simulink model "motor_stepper"  (R2018b)
settings: Solver=VariableStepAuto  StartTime=0.0  StopTime=2  FixedStep=0.001  MaxStep=0.001  RelTol=1e-3  EnableMultiTasking=on
libraries: fl_lib x27, nesl_utility x6, elec_lib x2, simulink x1
CloseFcn:
  | try,close(h1_elec_motor_stepper),end
  | clear h1_elec_motor_stepper
  | try,close(h2_elec_motor_stepper),end
  | clear h2_elec_motor_stepper
  | 
  | clear simlog_elec_motor_stepper
  | clear logsout_elec_motor_stepper
  | clear RPM2 tout
Description:
  | Stepper Motor with Control
  | 
  | Copyright 2008-2018 The MathWorks, Inc.
settings Model: Creator=MathWorks  LastModifiedBy=Administrator
settings DataIOCC: MaxDataPoints=10000  SaveFormat=Array  SignalLoggingName=logsout_elec_motor_stepper
settings OptimizationCC: ExpressionDepthLimit=2147483647  InitFltsAndDblsToZero=on  LifeSpan=inf
settings DebuggingCC: UnderspecifiedInitializationDetection=Classic  MergeDetectMultiDrivingBlocksExec=none  FcnCallInpInsideContextMsg=warning  StateNameClashWarn=warning  LibraryContextMissingDiagnostic=none  SFUnexpectedBacktrackingDiag=warning  SFNoUnconditionalDefaultTransitionDiag=warning  SFExecutionAtInitializationDiag=none
settings HardwareCC: ProdBitPerPointer=32  ProdBitPerSizeT=32  ProdBitPerPtrDiffT=32  ProdLargestAtomicFloat=None  ProdIntDivRoundTo=Undefined  ProdEndianess=Unspecified  ProdWordSize=32  ProdHWDeviceType=32-bit Generic
settings ModelReferenceCC: PropagateSignalLabelsOutOfModel=off
settings SFSimCC: SimUseLocalCustomCode=off
settings RTWCC: RTWUseLocalCustomCode=off
settings CodeAppCC: StateflowObjectComments=on
settings GRTTargetCC: TargetLangStandard=C89/C90 (ANSI)  GeneratePreprocessorConditionals=Disable all  CombineOutputUpdateFcns=off  GRTInterface=on
settings ConfigComp: CovScope=ReferencedModels  CovMetricSettings=dw  CovHtmlReporting=on  CovSaveCumulativeToWorkspaceVar=on  CovSaveSingleToWorkspaceVar=on  CovExternalEMLEnable=off  CovSFcnEnable=off
settings SimscapeCC: SimscapeLogType=all  SimscapeLogSimulationStatistics=on  SimscapeLogName=simlog_elec_motor_stepper  SimscapeLogDataHistory=10000

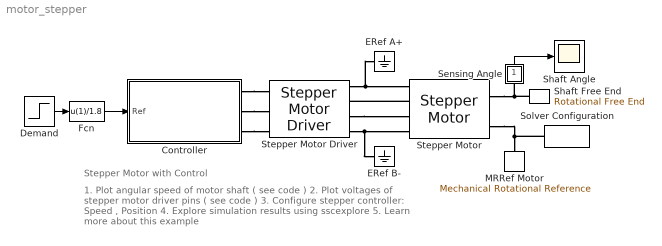
== system motor_stepper ==
  note: Stepper Motor with Control
  note: 1. Plot angular speed of motor shaft ( see code )
      | 2. Plot voltages of stepper motor driver pins ( see code )
      | 3. Configure stepper controller: Speed , Position
      | 4. Explore simulation results using sscexplore
      | 5. Learn more about this example
  Controller : Subsystem  VariantControlMode=Label  Variant=on  LabelModeActiveChoice=Position
      settings: AttributesFormatString=%<BlockChoice>
  Demand : Step  Before=10  After=0  SampleTime=0
  ERef A+ : fl_lib/Electrical/Electrical Elements/Electrical Reference
      settings: SourceProductName=Foundation Library
  ERef B- : fl_lib/Electrical/Electrical Elements/Electrical Reference
      settings: SourceProductName=Foundation Library
  Fcn : Fcn  Expr=u(1)/1.8
  MRRef Motor : fl_lib/Mechanical/Rotational Elements/Mechanical Rotational Reference
      settings: SourceProductName=Foundation Library
  Sensing Angle : Subsystem
      mask Display: disp('a')
  Shaft Angle : Scope
  Shaft Free End : fl_lib/Mechanical/Rotational Elements/Rotational Free End  w_specify=off  w_priority=None  w=0 rad/s  w_nominal_specify=off  w_nominal_unit=rad/s  w_nominal_value=1
      settings: SourceProductName=Foundation Library
  Solver Configuration : nesl_utility/Solver Configuration  PhysicalDomain=network_engine_domain  SubClassName=solver  LeftPortType=input  RightPortType=generic  Tones=[]  Harmonics=[]  SimulateNoise=off  Profile=off  UseLocalSampling=off  EnableSwitchedLinearOptims=on  FrequencyDomain=off  UseCCode=off  RelTol=0.001  AbsTol=1e-06  MinStep=1e-09  ToWorkspace=off  RevertToSquareIcSolve=off  NumHomotopyIterations=100  PhasorMode=off  PhasorModeNumHarmonics=1  DoDC=off  ResidualTolerance=1e-9  UseLocalSolver=off  LocalSolverChoice=NE_BACKWARD_EULER_ADVANCER  LocalSolverSampleTime=.001  DoFixedCost=off  MaxNonlinIter=3  MaxModeIter=2  LinearAlgebra=auto  EquationFormulation=NE_TIME_EF  DelaysMemoryBudget=1024  AutomaticFiltering=on  FilteringTimeConstant=0.001  PartitionStorageMethod=AS_NEEDED  PartitionMemoryBudget=1024
  Stepper Motor : elec_lib/Actuators & Drivers/Rotational Actuators/Stepper Motor  step_or_av=1  w_vec=[ 0 1000 3e+3 ] rpm  T_vec=[ 2 2 1 ] N*m  assert_if_slipping=0  J_total=1e-4 kg*m^2  max_step_rate=10 Hz  Ra=0.55 Ohm  La=0.0015 H  Km=0.19 N*m/A  Td=0 N*m  Rm=Inf Ohm  Step=1.8 deg  J=4.5e-05 kg*m^2  B=1e-02 N*m/(rad/s)  speed0=0 rpm  theta0=0 deg  alpha=[ 0.00393 0.00393 ] 1/K  Tmeas=25 degC  T_vec2=[ 1.7 1.7 0.85 ] N*m  Tmeas2=125 degC  half_stepping=0  thermal_masses=[ 100 100 ] J/K  initial_temperatures=[ 25 25 ] degC  rotor_thermal_mass=50 J/K  rotor_initial_temperature=25 degC  Rm_percent_rotor=90
      settings: SourceProductName=Simscape Electronics  SourceProductBaseCode=SN
  Stepper Motor Driver : elec_lib/Actuators & Drivers/Drivers/Stepper Motor Driver  step_or_av=1  step_rate_per_volt=10 Hz/V  Venable=2.5 V  Vreverse=2.5 V  Vm=5 V  half_stepping=0
      settings: SourceProductName=Simscape Electronics  SourceProductBaseCode=SN
  wires:
  Demand/1 -> Fcn/1
  Sensing Angle/1(theta) -> Shaft Angle/1
  Fcn/1 -> Controller/1(Ref)
  connections:
  Stepper Motor Driver/RConn1 -- Stepper Motor/LConn1 -- ERef A+/LConn1
  Stepper Motor/LConn2 -- Stepper Motor Driver/RConn2
  Stepper Motor Driver/RConn3 -- Stepper Motor/LConn3
  Stepper Motor Driver/RConn4 -- Stepper Motor/LConn4 -- ERef B-/LConn1
  Stepper Motor/RConn1 -- Shaft Free End/LConn1 -- Sensing Angle/LConn1
  Stepper Motor/RConn2 -- Solver Configuration/RConn1 -- MRRef Motor/LConn1
  Controller/RConn1 -- Stepper Motor Driver/LConn1
  Controller/RConn2 -- Stepper Motor Driver/LConn2
  Controller/RConn3 -- Stepper Motor Driver/LConn3

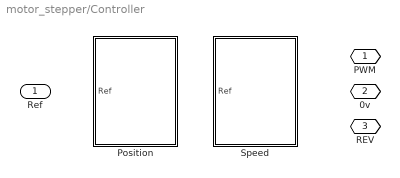
== system motor_stepper/Controller ==
  Ref : Inport
  Position : Subsystem  VariantControl=Position
  Speed : Subsystem  VariantControl=Speed
  PWM : PMIOPort  Side=Right
  0v : PMIOPort  Port=2  Side=Right
  REV : PMIOPort  Port=3  Side=Right

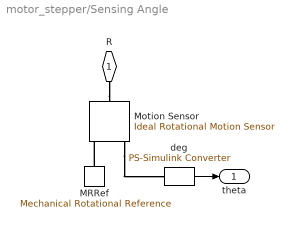
== system motor_stepper/Sensing Angle ==
  MRRef : fl_lib/Mechanical/Rotational Elements/Mechanical Rotational Reference
      settings: SourceProductName=Foundation Library
  Motion Sensor : fl_lib/Mechanical/Mechanical Sensors/Ideal Rotational Motion Sensor  offset=0 rad
      settings: SourceProductName=Foundation Library
  deg : nesl_utility/PS-Simulink Converter  PhysicalDomain=network_engine_domain  SubClassName=ps_output  LeftPortType=input  RightPortType=output  PseudoPeriodic=off  Frequencies=[]  Unit=deg  AffineConversion=off
  R : PMIOPort  Side=Left
  theta : Outport
  wires:
  deg/1 -> theta/1
  connections:
  R/RConn1 -- Motion Sensor/LConn1
  Motion Sensor/RConn3 -- deg/LConn1
  MRRef/LConn1 -- Motion Sensor/RConn1

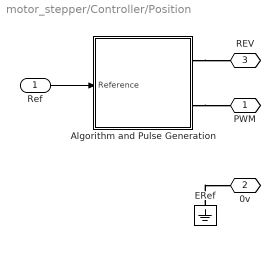
== system motor_stepper/Controller/Position ==
  Ref : Inport
  Algorithm and Pulse Generation : Subsystem
  ERef : fl_lib/Electrical/Electrical Elements/Electrical Reference
      settings: SourceProductName=Foundation Library
  PWM : PMIOPort  Side=Right
  0v : PMIOPort  Port=2  Side=Right
  REV : PMIOPort  Port=3  Side=Right
  wires:
  Ref/1 -> Algorithm and Pulse Generation/1(Reference)
  connections:
  Algorithm and Pulse Generation/RConn2 -- PWM/RConn1
  Algorithm and Pulse Generation/RConn1 -- REV/RConn1
  ERef/LConn1 -- 0v/RConn1

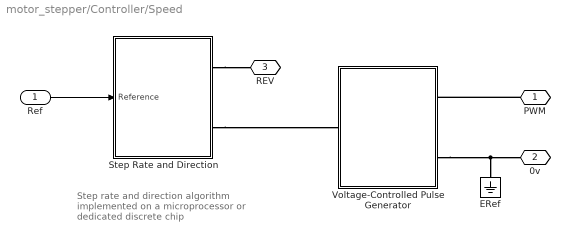
== system motor_stepper/Controller/Speed ==
  note: Step rate and direction algorithm implemented on a microprocessor or dedicated discrete chip
  Ref : Inport
  ERef : fl_lib/Electrical/Electrical Elements/Electrical Reference
      settings: SourceProductName=Foundation Library
  Step Rate and Direction : Subsystem
  Voltage-Controlled Pulse Generator : Subsystem
  PWM : PMIOPort  Side=Right
  0v : PMIOPort  Port=2  Side=Right
  REV : PMIOPort  Port=3  Side=Right
  wires:
  Ref/1 -> Step Rate and Direction/1(Reference)
  connections:
  PWM/RConn1 -- Voltage-Controlled Pulse Generator/RConn1
  Voltage-Controlled Pulse Generator/RConn2 -- 0v/RConn1 -- ERef/LConn1
  Step Rate and Direction/RConn1 -- REV/RConn1
  Step Rate and Direction/RConn2 -- Voltage-Controlled Pulse Generator/LConn1

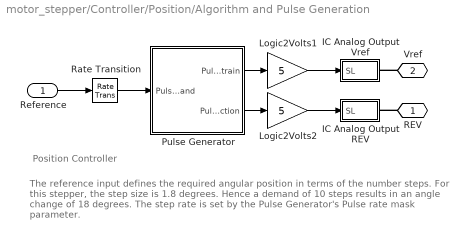
== system motor_stepper/Controller/Position/Algorithm and Pulse Generation ==
  note: The reference input defines the required angular position in terms of
      | the number steps. For this stepper, the step size is 1.8 degrees. Hence
      | a demand of 10 steps results in an angle change of 18 degrees.
      | The step rate is set by the Pulse Generator's Pulse rate mask parameter.
  note: Position Controller
  Reference : Inport
  IC Analog Output REV : Subsystem
  IC Analog Output Vref : Subsystem
  Logic2Volts1 : Gain  Gain=5
  Logic2Volts2 : Gain  Gain=5
  Pulse Generator : Subsystem  mask{f=20}
      mask prompts: f "Pulse rate"
  Rate Transition : RateTransition  Deterministic=off
  REV : PMIOPort  Side=Right
  Vref : PMIOPort  Port=2  Side=Right
  wires:
  Logic2Volts1/1 -> IC Analog Output Vref/1(SL)
  Pulse Generator/1(Pulse train) -> Logic2Volts1/1
  Reference/1 -> Rate Transition/1
  Logic2Volts2/1 -> IC Analog Output REV/1(SL)
  Pulse Generator/2(Pulse direction) -> Logic2Volts2/1
  Rate Transition/1 -> Pulse Generator/1(Pulse  demand)
  connections:
  Vref/RConn1 -- IC Analog Output Vref/RConn1
  REV/RConn1 -- IC Analog Output REV/RConn1

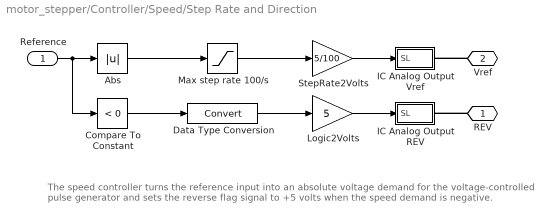
== system motor_stepper/Controller/Speed/Step Rate and Direction ==
  note: The speed controller turns the reference input into an absolute voltage demand for the
      | voltage-controlled pulse generator and sets the reverse flag signal to +5 volts when the
      | speed demand is negative.
  Reference : Inport
  Abs : Abs
  Compare To Constant : simulink/Logic and Bit Operations/Compare To Constant  relop=<  const=0  OutDataTypeStr=uint8  ZeroCross=off
  Data Type Conversion : DataTypeConversion
  IC Analog Output REV : Subsystem
  IC Analog Output Vref : Subsystem
  Logic2Volts : Gain  Gain=5
  Max step rate 100/s : Saturate  UpperLimit=100  LowerLimit=0
  StepRate2Volts : Gain  Gain=5/100
  REV : PMIOPort  Side=Right
  Vref : PMIOPort  Port=2  Side=Right
  wires:
  StepRate2Volts/1 -> IC Analog Output Vref/1(SL)
  Max step rate 100/s/1 -> StepRate2Volts/1
  Data Type Conversion/1 -> Logic2Volts/1
  Compare To Constant/1 -> Data Type Conversion/1
  Reference/1 -> Compare To Constant/1, Abs/1
  Abs/1 -> Max step rate 100/s/1
  Logic2Volts/1 -> IC Analog Output REV/1(SL)
  connections:
  REV/RConn1 -- IC Analog Output REV/RConn1
  Vref/RConn1 -- IC Analog Output Vref/RConn1

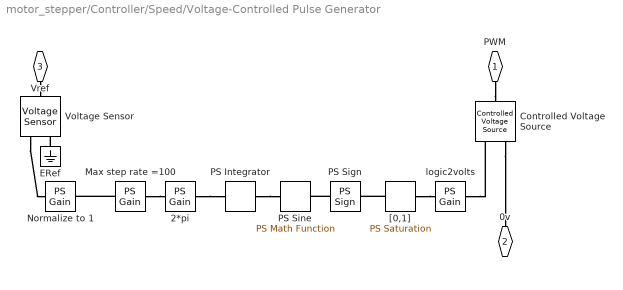
== system motor_stepper/Controller/Speed/Voltage-Controlled Pulse Generator ==
  2*pi : fl_lib/Physical Signals/Functions/PS Gain  gain=-2*pi
      settings: SourceProductName=Foundation Library
  Controlled Voltage Source : fl_lib/Electrical/Electrical Sources/Controlled Voltage Source
      settings: SourceProductName=Foundation Library
  ERef : fl_lib/Electrical/Electrical Elements/Electrical Reference
      settings: SourceProductName=Foundation Library
  Max step rate =100 : fl_lib/Physical Signals/Functions/PS Gain  gain=100
      settings: SourceProductName=Foundation Library
  Normalize to 1 : fl_lib/Physical Signals/Functions/PS Gain  gain=1/5
      settings: SourceProductName=Foundation Library
  PS Integrator : fl_lib/Physical Signals/Linear Operators/PS Integrator  x0=0
      settings: SourceProductName=Foundation Library
  PS Sign : fl_lib/Physical Signals/Nonlinear Operators/PS Sign
      settings: SourceProductName=Foundation Library
  PS Sine : fl_lib/Physical Signals/Functions/PS Math Function  fcn_choice=1
      settings: SourceProductName=Foundation Library
  Voltage Sensor : fl_lib/Electrical/Electrical Sensors/Voltage Sensor
      settings: SourceProductName=Foundation Library
  "[0,1]" : fl_lib/Physical Signals/Nonlinear Operators/PS Saturation  upper_limit=1  lower_limit=0
      settings: SourceProductName=Foundation Library
  logic2volts : fl_lib/Physical Signals/Functions/PS Gain  gain=5
      settings: SourceProductName=Foundation Library
  PWM : PMIOPort  Side=Right
  0v : PMIOPort  Port=2  Side=Right
  Vref : PMIOPort  Port=3  Side=Left
  connections:
  PWM/RConn1 -- Controlled Voltage Source/LConn1
  Controlled Voltage Source/RConn2 -- 0v/RConn1
  Vref/RConn1 -- Voltage Sensor/LConn1
  ERef/LConn1 -- Voltage Sensor/RConn2
  Voltage Sensor/RConn1 -- Normalize to 1/LConn1
  Max step rate =100/LConn1 -- Normalize to 1/RConn1
  Max step rate =100/RConn1 -- 2*pi/LConn1
  2*pi/RConn1 -- PS Integrator/LConn1
  PS Integrator/RConn1 -- PS Sine/LConn1
  PS Sign/LConn1 -- PS Sine/RConn1
  "[0,1]"/LConn1 -- PS Sign/RConn1
  "[0,1]"/RConn1 -- logic2volts/LConn1
  logic2volts/RConn1 -- Controlled Voltage Source/RConn1

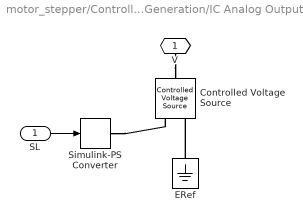
== system motor_stepper/Controller/Position/Algorithm and Pulse Generation/IC Analog Output REV ==
  SL : Inport
  Controlled Voltage Source : fl_lib/Electrical/Electrical Sources/Controlled Voltage Source
      settings: SourceProductName=Foundation Library
  ERef : fl_lib/Electrical/Electrical Elements/Electrical Reference
      settings: SourceProductName=Foundation Library
  Simulink-PS Converter : nesl_utility/Simulink-PS Converter  PhysicalDomain=network_engine_domain  SubClassName=ps_input  LeftPortType=input  RightPortType=output  PseudoPeriodic=off  Frequencies=[]  NoiseDistribution=none  NoiseParameters=[]  Unit=V  AffineConversion=off  FilteringAndDerivatives=zero  SimscapeFilterOrder=1  InputFilterTimeConstant=.001  UdotUserProvided=0
  V : PMIOPort  Side=Right
  wires:
  SL/1 -> Simulink-PS Converter/1
  connections:
  ERef/LConn1 -- Controlled Voltage Source/RConn2
  V/RConn1 -- Controlled Voltage Source/LConn1
  Simulink-PS Converter/RConn1 -- Controlled Voltage Source/RConn1

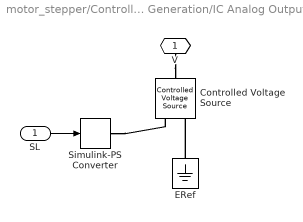
== system motor_stepper/Controller/Position/Algorithm and Pulse Generation/IC Analog Output Vref ==
  SL : Inport
  Controlled Voltage Source : fl_lib/Electrical/Electrical Sources/Controlled Voltage Source
      settings: SourceProductName=Foundation Library
  ERef : fl_lib/Electrical/Electrical Elements/Electrical Reference
      settings: SourceProductName=Foundation Library
  Simulink-PS Converter : nesl_utility/Simulink-PS Converter  PhysicalDomain=network_engine_domain  SubClassName=ps_input  LeftPortType=input  RightPortType=output  PseudoPeriodic=off  Frequencies=[]  NoiseDistribution=none  NoiseParameters=[]  Unit=V  AffineConversion=off  FilteringAndDerivatives=zero  SimscapeFilterOrder=1  InputFilterTimeConstant=.001  UdotUserProvided=0
  V : PMIOPort  Side=Right
  wires:
  SL/1 -> Simulink-PS Converter/1
  connections:
  Simulink-PS Converter/RConn1 -- Controlled Voltage Source/RConn1
  V/RConn1 -- Controlled Voltage Source/LConn1
  ERef/LConn1 -- Controlled Voltage Source/RConn2

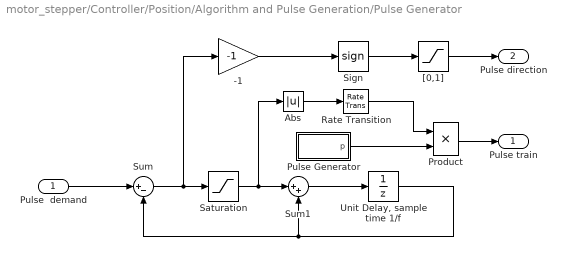
== system motor_stepper/Controller/Position/Algorithm and Pulse Generation/Pulse Generator ==
  Pulse  demand : Inport  SampleTime=1/f
  -1 : Gain  Gain=-1
  Abs : Abs
  Product : Product  SaturateOnIntegerOverflow=on  InputSameDT=on  OutDataTypeStr=Inherit: Same as first input
  Pulse Generator : Subsystem
  Rate Transition : RateTransition  Deterministic=off
  Saturation : Saturate  UpperLimit=1  LowerLimit=-1
  Sign : Signum
  Sum : Sum  Inputs=|+-
  Sum1 : Sum  Inputs=|++
  "Unit Delay, sample time 1/f" : UnitDelay  SampleTime=1/f
  "[0,1]" : Saturate  UpperLimit=1  LowerLimit=0
  Pulse train : Outport
  Pulse direction : Outport  Port=2
  wires:
  "[0,1]"/1 -> Pulse direction/1
  -1/1 -> Sign/1
  "Unit Delay, sample time 1/f"/1 -> Sum/2, Sum1/2
  Pulse  demand/1 -> Sum/1
  Sum/1 -> -1/1, Saturation/1
  Saturation/1 -> Sum1/1, Abs/1
  Sum1/1 -> "Unit Delay, sample time 1/f"/1
  Sign/1 -> "[0,1]"/1
  Product/1 -> Pulse train/1
  Abs/1 -> Rate Transition/1
  Pulse Generator/1(p) -> Product/2
  Rate Transition/1 -> Product/1

== system motor_stepper/Controller/Speed/Step Rate and Direction/IC Analog Output REV ==
  SL : Inport
  Controlled Voltage Source : fl_lib/Electrical/Electrical Sources/Controlled Voltage Source
      settings: SourceProductName=Foundation Library
  ERef : fl_lib/Electrical/Electrical Elements/Electrical Reference
      settings: SourceProductName=Foundation Library
  Simulink-PS Converter : nesl_utility/Simulink-PS Converter  PhysicalDomain=network_engine_domain  SubClassName=ps_input  LeftPortType=input  RightPortType=output  PseudoPeriodic=off  Frequencies=[]  NoiseDistribution=none  NoiseParameters=[]  Unit=V  AffineConversion=off  FilteringAndDerivatives=zero  SimscapeFilterOrder=1  InputFilterTimeConstant=.001  UdotUserProvided=0
  V : PMIOPort  Side=Right
  wires:
  SL/1 -> Simulink-PS Converter/1
  connections:
  Simulink-PS Converter/RConn1 -- Controlled Voltage Source/RConn1
  V/RConn1 -- Controlled Voltage Source/LConn1
  ERef/LConn1 -- Controlled Voltage Source/RConn2

== system motor_stepper/Controller/Speed/Step Rate and Direction/IC Analog Output Vref ==
  SL : Inport
  Controlled Voltage Source : fl_lib/Electrical/Electrical Sources/Controlled Voltage Source
      settings: SourceProductName=Foundation Library
  ERef : fl_lib/Electrical/Electrical Elements/Electrical Reference
      settings: SourceProductName=Foundation Library
  Simulink-PS Converter : nesl_utility/Simulink-PS Converter  PhysicalDomain=network_engine_domain  SubClassName=ps_input  LeftPortType=input  RightPortType=output  PseudoPeriodic=off  Frequencies=[]  NoiseDistribution=none  NoiseParameters=[]  Unit=V  AffineConversion=off  FilteringAndDerivatives=zero  SimscapeFilterOrder=1  InputFilterTimeConstant=.001  UdotUserProvided=0
  V : PMIOPort  Side=Right
  wires:
  SL/1 -> Simulink-PS Converter/1
  connections:
  ERef/LConn1 -- Controlled Voltage Source/RConn2
  V/RConn1 -- Controlled Voltage Source/LConn1
  Simulink-PS Converter/RConn1 -- Controlled Voltage Source/RConn1

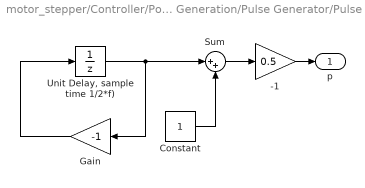
== system motor_stepper/Controller/Position/Algorithm and Pulse Generation/Pulse Generator/Pulse Generator ==
  -1 : Gain  Gain=0.5
  Constant : Constant  SampleTime=1/(2*f)
  Gain : Gain  Gain=-1
  Sum : Sum  Inputs=|++
  "Unit Delay, sample time 1/2*f)" : UnitDelay  InitialCondition=-1  SampleTime=1/(2*f)
  p : Outport
  wires:
  "Unit Delay, sample time 1/2*f)"/1 -> Gain/1, Sum/1
  Gain/1 -> "Unit Delay, sample time 1/2*f)"/1
  Constant/1 -> Sum/2
  Sum/1 -> -1/1
  -1/1 -> p/1
